simulink model "Copy_4_of_baseModel"  (R2019a)
settings: Solver=ode1  StartTime=0.0  StopTime=2.5  FixedStep=Ts_Power  RelTol=1e-3
PostLoadFcn:
  | %% Init for wind PnO models - global system parameters
  | OVERRIDE_SSN_MEMORY_LIMIT=1;
  | Ts=50e-6;
  | % Ts=50e-10;
  | Ts_Power=Ts;
  | Ts_Control=2*Ts;
  | freq = 50;
  | Fnom=freq;
  | Vac=400e3;
InitFcn:
  | %% Init for wind PnO models - global system parameters
  | OVERRIDE_SSN_MEMORY_LIMIT=1;
  | Ts=50e-6;
  | % Ts=50e-10;
  | Ts_Power=Ts;
  | Ts_Control=2*Ts;
  | freq = 50;
  | Fnom=freq;
  | Vac=225e3;
values from neighbouring files (symbols this model uses):
  ohl_posCap = (0.01e-006)*12    (= 1.2e-07)    [variable.m]
  ohl_posInd = (1.15e-3)/12    (= 9.58333333333e-05)    [variable.m]
  ohl_posR = 0.069/12    (= 0.00575)    [variable.m]
  ohl_zeroCap = (0.004e-006)*12    (= 4.8e-08)    [variable.m]
  ohl_zeroInd = (2.86e-3)/12    (= 0.000238333333333)    [variable.m]
  ohl_zeroR = 0.1725/12    (= 0.014375)    [variable.m]
  sub_posCap = sub_posCap*6    (= 9.6e-07)    [variable.m]
  sub_posInd = sub_posInd/6    (= 0.000233333333333)    [variable.m]
  sub_posR = sub_posR/6    (= 0.006)    [variable.m]
  sub_zeroCap = sub_zeroCap*6    (= 3.84e-07)    [variable.m]
  sub_zeroInd = sub_zeroInd/6    (= 0.000583333333333)    [variable.m]
  sub_zeroR = sub_zeroR/6    (= 0.015)    [variable.m]
  transfo_L1 = 0.05999374    [variable.m]
  transfo_L2 = 0.05999374    [variable.m]
  transfo_R1 = 0.000866667    [variable.m]
  transfo_R2 = 0.00086667    [variable.m]
undefined symbols (not defined in the file or in its folder): D1, D11, Delta, den, DiscIntNeverNeededParam, dx, find_system, gcbh, num, out_Buses, out_WindFarms, sps_rtmsupport
libraries: powerlib x172, simulink x80, powerlib_meascontrol x80, elements x52, eeSinusoidalMeasurement x44, simulink_extras x40, spsVIMeasurementModel x33, eePowerMeasurement x14
(part 10 of 22)

== system Copy_4_of_baseModel/SM_WT1/Differential Element 1/Main Protection (Current Differential)/Current Differential Protection for Phase C ==
  Ilocal : Inport
  Iremote : Inport  Port=2
  Icomp : Inport  Port=3
  " " : elements/   fo=Freq  window_size=40  harmonic=[1 2 3 4 5]
  " 1" : elements/   fo=Freq  window_size=40  harmonic=[1 2 3 4 5]
  Comparing Current at Master Station : Sum  Inputs=+-  SaturateOnIntegerOverflow=on  InputSameDT=on  OutDataTypeStr=Inherit: Same as first input
  Comparision Scheme : Subsystem
  DAB4 : Subsystem  mask(Data Adquisition Board){filter=off, approx=Bessel, order=2, numerator=[], denominator=[], freq=180, resdis=off, vertres=12, xmax=10, winsize=40, G=1.0, fs=Freq*40}
      mask prompts: filter "Disable Analog Filter"; approx "Filter approximation"; numerator "Free expression filter: numerator(descending order of s)"; denominator "Free expression filter: denominator:"; freq "Cut-off frequency"; resdis "Disable Vertical Resolution"; vertres "Vertical Resolution: No. of bits"; xmax "Vertical Resolution: signal range"; winsize "Window size"; G "Gain"; fs "Sampling frequency"
      mask help: Performs analog filtering, signal conditioning and sampling. A single signal is the input, a buffer with the signal samples is the output. The options include analog filter enable/disable switch, type, order and cut-off frequency of the analog filter, conditioning gain, sampling frequency, number of bits, the length of the buffer.
      mask init:
      | dab1
      mask TypeOptions approx: Bessel | Tschebyscheff | Butterworth | free expression
      mask TypeOptions order: 2 | 3 | 4
      mask TypeOptions vertres: 8 | 12 | 16
      mask Display: disp('DAB')
  DAB8 : Subsystem  mask(Data Adquisition Board){filter=off, approx=Bessel, order=2, numerator=[], denominator=[], freq=180, resdis=off, vertres=12, xmax=10, winsize=40, G=1.0, fs=Freq*40}
      mask prompts: filter "Disable Analog Filter"; approx "Filter approximation"; numerator "Free expression filter: numerator(descending order of s)"; denominator "Free expression filter: denominator:"; freq "Cut-off frequency"; resdis "Disable Vertical Resolution"; vertres "Vertical Resolution: No. of bits"; xmax "Vertical Resolution: signal range"; winsize "Window size"; G "Gain"; fs "Sampling frequency"
      mask help: Performs analog filtering, signal conditioning and sampling. A single signal is the input, a buffer with the signal samples is the output. The options include analog filter enable/disable switch, type, order and cut-off frequency of the analog filter, conditioning gain, sampling frequency, number of bits, the length of the buffer.
      mask init:
      | dab1
      mask TypeOptions approx: Bessel | Tschebyscheff | Butterworth | free expression
      mask TypeOptions order: 2 | 3 | 4
      mask TypeOptions vertres: 8 | 12 | 16
      mask Display: disp('DAB')
  Degrees to Radians : simulink_extras/Transformations/Degrees to Radians
  Degrees to Radians1 : simulink_extras/Transformations/Degrees to Radians
  Demux1 : Demux  Outputs=2
  Demux2 : Demux  Outputs=2
  Gain : Gain  SaturateOnIntegerOverflow=on  OutDataTypeStr=Inherit: Same as input  ParamDataTypeStr=Inherit: Same as input
  Gain1 : Gain  SaturateOnIntegerOverflow=on  OutDataTypeStr=Inherit: Same as input  ParamDataTypeStr=Inherit: Same as input
  Magnitude-Angle to Complex : MagnitudeAngleToComplex
  Magnitude-Angle to Complex1 : MagnitudeAngleToComplex
  Mux1 : Mux
  Mux2 : Mux
  Terminator1 : Terminator
  Terminator2 : Terminator
  Trip : Outport  InitialOutput=0  VectorParamsAs1DForOutWhenUnconnected=on
  wires:
  Gain1/1 -> Comparing Current at Master Station/2
  " 1"/2 -> Mux2/1
  " 1"/4 -> Mux2/3
  " 1"/3 -> Mux2/2
  Mux2/1 -> Terminator2/1
  Gain/1 -> DAB8/1(a)
  Iremote/1 -> Gain/1
  " 1"/1 -> Demux2/1
  DAB8/1(d) -> " 1"/1
  Magnitude-Angle to Complex1/1 -> Comparision Scheme/2(I_Master)
  Demux2/2 -> Degrees to Radians/1
  Degrees to Radians/1 -> Magnitude-Angle to Complex1/2
  Demux2/1 -> Magnitude-Angle to Complex1/1
  " "/5 -> Mux1/4
  " "/4 -> Mux1/3
  " "/3 -> Mux1/2
  " "/2 -> Mux1/1
  Mux1/1 -> Terminator1/1
  " "/1 -> Demux1/1
  Comparision Scheme/1(Pickup) -> Trip/1
  DAB4/1(d) -> " "/1
  Ilocal/1 -> DAB4/1(a)
  Magnitude-Angle to Complex/1 -> Comparing Current at Master Station/1
  Icomp/1 -> Gain1/1
  Demux1/2 -> Degrees to Radians1/1
  Degrees to Radians1/1 -> Magnitude-Angle to Complex/2
  Comparing Current at Master Station/1 -> Comparision Scheme/1(I_Slave)
  " 1"/5 -> Mux2/4
  Demux1/1 -> Magnitude-Angle to Complex/1

== system Copy_4_of_baseModel/SM_WT1/Differential Element 2/Main Protection (Current Differential)/Charging Current Compensation phase A ==
  VA : Inport
  VB : Inport  Port=2
  VC : Inport  Port=3
  " 5" : elements/   fo=Freq  window_size=40  harmonic=[1 2 3 4 5]
  " 6" : elements/   fo=Freq  window_size=40  harmonic=[1 2 3 4 5]
  " 7" : elements/   fo=Freq  window_size=40  harmonic=[1 2 3 4 5]
  *2 : Gain  Gain=2  SaturateOnIntegerOverflow=on  OutDataTypeStr=Inherit: Same as input  ParamDataTypeStr=Inherit: Same as input
  Compensating Current : Sum  SaturateOnIntegerOverflow=on  InputSameDT=on  OutDataTypeStr=Inherit: Same as first input
  Cpg : Gain  Gain=Cpg  SaturateOnIntegerOverflow=on  OutDataTypeStr=Inherit: Same as input  ParamDataTypeStr=Inherit: Same as input
  Cpp : Gain  Gain=Cpp  SaturateOnIntegerOverflow=on  OutDataTypeStr=Inherit: Same as input  ParamDataTypeStr=Inherit: Same as input
  DAB5 : Subsystem  mask(Data Adquisition Board){filter=off, approx=Bessel, order=2, numerator=[], denominator=[], freq=180, resdis=off, vertres=12, xmax=10, winsize=40, G=1.0, fs=Freq*40}
      mask prompts: filter "Disable Analog Filter"; approx "Filter approximation"; numerator "Free expression filter: numerator(descending order of s)"; denominator "Free expression filter: denominator:"; freq "Cut-off frequency"; resdis "Disable Vertical Resolution"; vertres "Vertical Resolution: No. of bits"; xmax "Vertical Resolution: signal range"; winsize "Window size"; G "Gain"; fs "Sampling frequency"
      mask help: Performs analog filtering, signal conditioning and sampling. A single signal is the input, a buffer with the signal samples is the output. The options include analog filter enable/disable switch, type, order and cut-off frequency of the analog filter, conditioning gain, sampling frequency, number of bits, the length of the buffer.
      mask init:
      | dab1
      mask TypeOptions approx: Bessel | Tschebyscheff | Butterworth | free expression
      mask TypeOptions order: 2 | 3 | 4
      mask TypeOptions vertres: 8 | 12 | 16
      mask Display: disp('DAB')
  DAB6 : Subsystem  mask(Data Adquisition Board){filter=off, approx=Bessel, order=2, numerator=[], denominator=[], freq=180, resdis=off, vertres=12, xmax=10, winsize=40, G=1.0, fs=Freq*40}
      mask prompts: filter "Disable Analog Filter"; approx "Filter approximation"; numerator "Free expression filter: numerator(descending order of s)"; denominator "Free expression filter: denominator:"; freq "Cut-off frequency"; resdis "Disable Vertical Resolution"; vertres "Vertical Resolution: No. of bits"; xmax "Vertical Resolution: signal range"; winsize "Window size"; G "Gain"; fs "Sampling frequency"
      mask help: Performs analog filtering, signal conditioning and sampling. A single signal is the input, a buffer with the signal samples is the output. The options include analog filter enable/disable switch, type, order and cut-off frequency of the analog filter, conditioning gain, sampling frequency, number of bits, the length of the buffer.
      mask init:
      | dab1
      mask TypeOptions approx: Bessel | Tschebyscheff | Butterworth | free expression
      mask TypeOptions order: 2 | 3 | 4
      mask TypeOptions vertres: 8 | 12 | 16
      mask Display: disp('DAB')
  DAB7 : Subsystem  mask(Data Adquisition Board){filter=off, approx=Bessel, order=2, numerator=[], denominator=[], freq=180, resdis=off, vertres=12, xmax=10, winsize=40, G=1.0, fs=Freq*40}
      mask prompts: filter "Disable Analog Filter"; approx "Filter approximation"; numerator "Free expression filter: numerator(descending order of s)"; denominator "Free expression filter: denominator:"; freq "Cut-off frequency"; resdis "Disable Vertical Resolution"; vertres "Vertical Resolution: No. of bits"; xmax "Vertical Resolution: signal range"; winsize "Window size"; G "Gain"; fs "Sampling frequency"
      mask help: Performs analog filtering, signal conditioning and sampling. A single signal is the input, a buffer with the signal samples is the output. The options include analog filter enable/disable switch, type, order and cut-off frequency of the analog filter, conditioning gain, sampling frequency, number of bits, the length of the buffer.
      mask init:
      | dab1
      mask TypeOptions approx: Bessel | Tschebyscheff | Butterworth | free expression
      mask TypeOptions order: 2 | 3 | 4
      mask TypeOptions vertres: 8 | 12 | 16
      mask Display: disp('DAB')
  Degrees to Radians1 : simulink_extras/Transformations/Degrees to Radians
  Degrees to Radians2 : simulink_extras/Transformations/Degrees to Radians
  Degrees to Radians3 : simulink_extras/Transformations/Degrees to Radians
  Demux : Demux  Outputs=2
  Demux1 : Demux  Outputs=2
  Demux2 : Demux  Outputs=2
  Derivative : Derivative
  Derivative1 : Derivative
  Derivative2 : Derivative
  Magnitude-Angle to Complex : MagnitudeAngleToComplex
  Magnitude-Angle to Complex1 : MagnitudeAngleToComplex
  Magnitude-Angle to Complex2 : MagnitudeAngleToComplex
  Mux : Mux  Inputs=12
  Terminator : Terminator
  sum : Sum  Inputs=+--  SaturateOnIntegerOverflow=on  InputSameDT=on  OutDataTypeStr=Inherit: Same as first input
  Icomp : Outport  VectorParamsAs1DForOutWhenUnconnected=on
  wires:
  " 5"/1 -> Demux2/1
  Demux1/2 -> Degrees to Radians2/1
  Demux1/1 -> Magnitude-Angle to Complex1/1
  " 7"/1 -> Demux/1
  Derivative1/1 -> DAB6/1(a)
  DAB6/1(d) -> " 6"/1
  " 6"/1 -> Demux1/1
  VB/1 -> Derivative1/1
  Mux/1 -> Terminator/1
  " 5"/5 -> Mux/4
  Derivative/1 -> DAB5/1(a)
  DAB5/1(d) -> " 5"/1
  Cpg/1 -> Compensating Current/1
  VA/1 -> Derivative/1
  " 5"/2 -> Mux/1
  " 5"/3 -> Mux/2
  " 5"/4 -> Mux/3
  sum/1 -> Cpp/1
  Compensating Current/1 -> Icomp/1
  *2/1 -> sum/1
  Cpp/1 -> Compensating Current/2
  Derivative2/1 -> DAB7/1(a)
  DAB7/1(d) -> " 7"/1
  VC/1 -> Derivative2/1
  " 7"/2 -> Mux/9
  " 7"/3 -> Mux/10
  " 7"/4 -> Mux/11
  " 7"/5 -> Mux/12
  " 6"/2 -> Mux/5
  " 6"/3 -> Mux/6
  " 6"/4 -> Mux/7
  " 6"/5 -> Mux/8
  Demux2/1 -> Magnitude-Angle to Complex/1
  Magnitude-Angle to Complex/1 -> *2/1, Cpg/1
  Magnitude-Angle to Complex1/1 -> sum/2
  Demux/1 -> Magnitude-Angle to Complex2/1
  Magnitude-Angle to Complex2/1 -> sum/3
  Demux/2 -> Degrees to Radians1/1
  Degrees to Radians1/1 -> Magnitude-Angle to Complex2/2
  Degrees to Radians2/1 -> Magnitude-Angle to Complex1/2
  Demux2/2 -> Degrees to Radians3/1
  Degrees to Radians3/1 -> Magnitude-Angle to Complex/2

== system Copy_4_of_baseModel/SM_WT1/Differential Element 2/Main Protection (Current Differential)/Charging Current Compensation phase B ==
  VA : Inport
  VB : Inport  Port=2
  VC : Inport  Port=3
  " 5" : elements/   fo=Freq  window_size=40  harmonic=[1 2 3 4 5]
  " 6" : elements/   fo=Freq  window_size=40  harmonic=[1 2 3 4 5]
  " 7" : elements/   fo=Freq  window_size=40  harmonic=[1 2 3 4 5]
  *2 : Gain  Gain=2  SaturateOnIntegerOverflow=on  OutDataTypeStr=Inherit: Same as input  ParamDataTypeStr=Inherit: Same as input
  Compensating Current : Sum  SaturateOnIntegerOverflow=on  InputSameDT=on  OutDataTypeStr=Inherit: Same as first input
  Cpg : Gain  Gain=Cpg  SaturateOnIntegerOverflow=on  OutDataTypeStr=Inherit: Same as input  ParamDataTypeStr=Inherit: Same as input
  Cpp : Gain  Gain=Cpp  SaturateOnIntegerOverflow=on  OutDataTypeStr=Inherit: Same as input  ParamDataTypeStr=Inherit: Same as input
  DAB5 : Subsystem  mask(Data Adquisition Board){filter=off, approx=Bessel, order=2, numerator=[], denominator=[], freq=180, resdis=off, vertres=12, xmax=10, winsize=40, G=1.0, fs=Freq*40}
      mask prompts: filter "Disable Analog Filter"; approx "Filter approximation"; numerator "Free expression filter: numerator(descending order of s)"; denominator "Free expression filter: denominator:"; freq "Cut-off frequency"; resdis "Disable Vertical Resolution"; vertres "Vertical Resolution: No. of bits"; xmax "Vertical Resolution: signal range"; winsize "Window size"; G "Gain"; fs "Sampling frequency"
      mask help: Performs analog filtering, signal conditioning and sampling. A single signal is the input, a buffer with the signal samples is the output. The options include analog filter enable/disable switch, type, order and cut-off frequency of the analog filter, conditioning gain, sampling frequency, number of bits, the length of the buffer.
      mask init:
      | dab1
      mask TypeOptions approx: Bessel | Tschebyscheff | Butterworth | free expression
      mask TypeOptions order: 2 | 3 | 4
      mask TypeOptions vertres: 8 | 12 | 16
      mask Display: disp('DAB')
  DAB6 : Subsystem  mask(Data Adquisition Board){filter=off, approx=Bessel, order=2, numerator=[], denominator=[], freq=180, resdis=off, vertres=12, xmax=10, winsize=40, G=1.0, fs=Freq*40}
      mask prompts: filter "Disable Analog Filter"; approx "Filter approximation"; numerator "Free expression filter: numerator(descending order of s)"; denominator "Free expression filter: denominator:"; freq "Cut-off frequency"; resdis "Disable Vertical Resolution"; vertres "Vertical Resolution: No. of bits"; xmax "Vertical Resolution: signal range"; winsize "Window size"; G "Gain"; fs "Sampling frequency"
      mask help: Performs analog filtering, signal conditioning and sampling. A single signal is the input, a buffer with the signal samples is the output. The options include analog filter enable/disable switch, type, order and cut-off frequency of the analog filter, conditioning gain, sampling frequency, number of bits, the length of the buffer.
      mask init:
      | dab1
      mask TypeOptions approx: Bessel | Tschebyscheff | Butterworth | free expression
      mask TypeOptions order: 2 | 3 | 4
      mask TypeOptions vertres: 8 | 12 | 16
      mask Display: disp('DAB')
  DAB7 : Subsystem  mask(Data Adquisition Board){filter=off, approx=Bessel, order=2, numerator=[], denominator=[], freq=180, resdis=off, vertres=12, xmax=10, winsize=40, G=1.0, fs=Freq*40}
      mask prompts: filter "Disable Analog Filter"; approx "Filter approximation"; numerator "Free expression filter: numerator(descending order of s)"; denominator "Free expression filter: denominator:"; freq "Cut-off frequency"; resdis "Disable Vertical Resolution"; vertres "Vertical Resolution: No. of bits"; xmax "Vertical Resolution: signal range"; winsize "Window size"; G "Gain"; fs "Sampling frequency"
      mask help: Performs analog filtering, signal conditioning and sampling. A single signal is the input, a buffer with the signal samples is the output. The options include analog filter enable/disable switch, type, order and cut-off frequency of the analog filter, conditioning gain, sampling frequency, number of bits, the length of the buffer.
      mask init:
      | dab1
      mask TypeOptions approx: Bessel | Tschebyscheff | Butterworth | free expression
      mask TypeOptions order: 2 | 3 | 4
      mask TypeOptions vertres: 8 | 12 | 16
      mask Display: disp('DAB')
  Degrees to Radians1 : simulink_extras/Transformations/Degrees to Radians
  Degrees to Radians2 : simulink_extras/Transformations/Degrees to Radians
  Degrees to Radians3 : simulink_extras/Transformations/Degrees to Radians
  Demux : Demux  Outputs=2
  Demux1 : Demux  Outputs=2
  Demux2 : Demux  Outputs=2
  Derivative : Derivative
  Derivative1 : Derivative
  Derivative2 : Derivative
  Magnitude-Angle to Complex : MagnitudeAngleToComplex
  Magnitude-Angle to Complex1 : MagnitudeAngleToComplex
  Magnitude-Angle to Complex2 : MagnitudeAngleToComplex
  Mux : Mux  Inputs=12
  Terminator : Terminator
  sum : Sum  Inputs=+--  SaturateOnIntegerOverflow=on  InputSameDT=on  OutDataTypeStr=Inherit: Same as first input
  Icomp : Outport  VectorParamsAs1DForOutWhenUnconnected=on
  wires:
  VA/1 -> Derivative1/1
  VB/1 -> Derivative/1
  " 5"/1 -> Demux2/1
  Demux1/2 -> Degrees to Radians2/1
  Demux1/1 -> Magnitude-Angle to Complex1/1
  " 7"/1 -> Demux/1
  Derivative1/1 -> DAB6/1(a)
  DAB6/1(d) -> " 6"/1
  " 6"/1 -> Demux1/1
  Mux/1 -> Terminator/1
  " 5"/5 -> Mux/4
  Derivative/1 -> DAB5/1(a)
  DAB5/1(d) -> " 5"/1
  Cpg/1 -> Compensating Current/1
  " 5"/2 -> Mux/1
  " 5"/3 -> Mux/2
  " 5"/4 -> Mux/3
  sum/1 -> Cpp/1
  Compensating Current/1 -> Icomp/1
  *2/1 -> sum/1
  Cpp/1 -> Compensating Current/2
  Derivative2/1 -> DAB7/1(a)
  DAB7/1(d) -> " 7"/1
  VC/1 -> Derivative2/1
  " 7"/2 -> Mux/9
  " 7"/3 -> Mux/10
  " 7"/4 -> Mux/11
  " 7"/5 -> Mux/12
  " 6"/2 -> Mux/5
  " 6"/3 -> Mux/6
  " 6"/4 -> Mux/7
  " 6"/5 -> Mux/8
  Demux2/1 -> Magnitude-Angle to Complex/1
  Magnitude-Angle to Complex/1 -> *2/1, Cpg/1
  Magnitude-Angle to Complex1/1 -> sum/2
  Demux/1 -> Magnitude-Angle to Complex2/1
  Magnitude-Angle to Complex2/1 -> sum/3
  Demux/2 -> Degrees to Radians1/1
  Degrees to Radians1/1 -> Magnitude-Angle to Complex2/2
  Degrees to Radians2/1 -> Magnitude-Angle to Complex1/2
  Demux2/2 -> Degrees to Radians3/1
  Degrees to Radians3/1 -> Magnitude-Angle to Complex/2

== system Copy_4_of_baseModel/SM_WT1/Differential Element 2/Main Protection (Current Differential)/Charging Current Compensation phase C ==
  VA : Inport
  VB : Inport  Port=2
  VC : Inport  Port=3
  " 5" : elements/   fo=Freq  window_size=40  harmonic=[1 2 3 4 5]
  " 6" : elements/   fo=Freq  window_size=40  harmonic=[1 2 3 4 5]
  " 7" : elements/   fo=Freq  window_size=40  harmonic=[1 2 3 4 5]
  *2 : Gain  Gain=2  SaturateOnIntegerOverflow=on  OutDataTypeStr=Inherit: Same as input  ParamDataTypeStr=Inherit: Same as input
  Compensating Current : Sum  SaturateOnIntegerOverflow=on  InputSameDT=on  OutDataTypeStr=Inherit: Same as first input
  Cpg : Gain  Gain=Cpg  SaturateOnIntegerOverflow=on  OutDataTypeStr=Inherit: Same as input  ParamDataTypeStr=Inherit: Same as input
  Cpp : Gain  Gain=Cpp  SaturateOnIntegerOverflow=on  OutDataTypeStr=Inherit: Same as input  ParamDataTypeStr=Inherit: Same as input
  DAB5 : Subsystem  mask(Data Adquisition Board){filter=off, approx=Bessel, order=2, numerator=[], denominator=[], freq=180, resdis=off, vertres=12, xmax=10, winsize=40, G=1.0, fs=Freq*40}
      mask prompts: filter "Disable Analog Filter"; approx "Filter approximation"; numerator "Free expression filter: numerator(descending order of s)"; denominator "Free expression filter: denominator:"; freq "Cut-off frequency"; resdis "Disable Vertical Resolution"; vertres "Vertical Resolution: No. of bits"; xmax "Vertical Resolution: signal range"; winsize "Window size"; G "Gain"; fs "Sampling frequency"
      mask help: Performs analog filtering, signal conditioning and sampling. A single signal is the input, a buffer with the signal samples is the output. The options include analog filter enable/disable switch, type, order and cut-off frequency of the analog filter, conditioning gain, sampling frequency, number of bits, the length of the buffer.
      mask init:
      | dab1
      mask TypeOptions approx: Bessel | Tschebyscheff | Butterworth | free expression
      mask TypeOptions order: 2 | 3 | 4
      mask TypeOptions vertres: 8 | 12 | 16
      mask Display: disp('DAB')
  DAB6 : Subsystem  mask(Data Adquisition Board){filter=off, approx=Bessel, order=2, numerator=[], denominator=[], freq=180, resdis=off, vertres=12, xmax=10, winsize=40, G=1.0, fs=Freq*40}
      mask prompts: filter "Disable Analog Filter"; approx "Filter approximation"; numerator "Free expression filter: numerator(descending order of s)"; denominator "Free expression filter: denominator:"; freq "Cut-off frequency"; resdis "Disable Vertical Resolution"; vertres "Vertical Resolution: No. of bits"; xmax "Vertical Resolution: signal range"; winsize "Window size"; G "Gain"; fs "Sampling frequency"
      mask help: Performs analog filtering, signal conditioning and sampling. A single signal is the input, a buffer with the signal samples is the output. The options include analog filter enable/disable switch, type, order and cut-off frequency of the analog filter, conditioning gain, sampling frequency, number of bits, the length of the buffer.
      mask init:
      | dab1
      mask TypeOptions approx: Bessel | Tschebyscheff | Butterworth | free expression
      mask TypeOptions order: 2 | 3 | 4
      mask TypeOptions vertres: 8 | 12 | 16
      mask Display: disp('DAB')
  DAB7 : Subsystem  mask(Data Adquisition Board){filter=off, approx=Bessel, order=2, numerator=[], denominator=[], freq=180, resdis=off, vertres=12, xmax=10, winsize=40, G=1.0, fs=Freq*40}
      mask prompts: filter "Disable Analog Filter"; approx "Filter approximation"; numerator "Free expression filter: numerator(descending order of s)"; denominator "Free expression filter: denominator:"; freq "Cut-off frequency"; resdis "Disable Vertical Resolution"; vertres "Vertical Resolution: No. of bits"; xmax "Vertical Resolution: signal range"; winsize "Window size"; G "Gain"; fs "Sampling frequency"
      mask help: Performs analog filtering, signal conditioning and sampling. A single signal is the input, a buffer with the signal samples is the output. The options include analog filter enable/disable switch, type, order and cut-off frequency of the analog filter, conditioning gain, sampling frequency, number of bits, the length of the buffer.
      mask init:
      | dab1
      mask TypeOptions approx: Bessel | Tschebyscheff | Butterworth | free expression
      mask TypeOptions order: 2 | 3 | 4
      mask TypeOptions vertres: 8 | 12 | 16
      mask Display: disp('DAB')
  Degrees to Radians1 : simulink_extras/Transformations/Degrees to Radians
  Degrees to Radians2 : simulink_extras/Transformations/Degrees to Radians
  Degrees to Radians3 : simulink_extras/Transformations/Degrees to Radians
  Demux : Demux  Outputs=2
  Demux1 : Demux  Outputs=2
  Demux2 : Demux  Outputs=2
  Derivative : Derivative
  Derivative1 : Derivative
  Derivative2 : Derivative
  Magnitude-Angle to Complex : MagnitudeAngleToComplex
  Magnitude-Angle to Complex1 : MagnitudeAngleToComplex
  Magnitude-Angle to Complex2 : MagnitudeAngleToComplex
  Mux : Mux  Inputs=12
  Terminator : Terminator
  sum : Sum  Inputs=+--  SaturateOnIntegerOverflow=on  InputSameDT=on  OutDataTypeStr=Inherit: Same as first input
  Icomp : Outport  VectorParamsAs1DForOutWhenUnconnected=on
  wires:
  VA/1 -> Derivative2/1
  VC/1 -> Derivative/1
  " 5"/1 -> Demux2/1
  Demux1/2 -> Degrees to Radians2/1
  Demux1/1 -> Magnitude-Angle to Complex1/1
  " 7"/1 -> Demux/1
  Derivative1/1 -> DAB6/1(a)
  DAB6/1(d) -> " 6"/1
  " 6"/1 -> Demux1/1
  VB/1 -> Derivative1/1
  Mux/1 -> Terminator/1
  " 5"/5 -> Mux/4
  Derivative/1 -> DAB5/1(a)
  DAB5/1(d) -> " 5"/1
  Cpg/1 -> Compensating Current/1
  " 5"/2 -> Mux/1
  " 5"/3 -> Mux/2
  " 5"/4 -> Mux/3
  sum/1 -> Cpp/1
  Compensating Current/1 -> Icomp/1
  *2/1 -> sum/1
  Cpp/1 -> Compensating Current/2
  Derivative2/1 -> DAB7/1(a)
  DAB7/1(d) -> " 7"/1
  " 7"/2 -> Mux/9
  " 7"/3 -> Mux/10
  " 7"/4 -> Mux/11
  " 7"/5 -> Mux/12
  " 6"/2 -> Mux/5
  " 6"/3 -> Mux/6
  " 6"/4 -> Mux/7
  " 6"/5 -> Mux/8
  Demux2/1 -> Magnitude-Angle to Complex/1
  Magnitude-Angle to Complex/1 -> *2/1, Cpg/1
  Magnitude-Angle to Complex1/1 -> sum/2
  Demux/1 -> Magnitude-Angle to Complex2/1
  Magnitude-Angle to Complex2/1 -> sum/3
  Demux/2 -> Degrees to Radians1/1
  Degrees to Radians1/1 -> Magnitude-Angle to Complex2/2
  Degrees to Radians2/1 -> Magnitude-Angle to Complex1/2
  Demux2/2 -> Degrees to Radians3/1
  Degrees to Radians3/1 -> Magnitude-Angle to Complex/2

== system Copy_4_of_baseModel/SM_WT1/Differential Element 2/Main Protection (Current Differential)/Current Differential Protection for Phase A ==
  Ilocal : Inport
  Iremote : Inport  Port=2
  Icomp : Inport  Port=3
  " " : elements/   fo=Freq  window_size=40  harmonic=[1 2 3 4 5]
  " 1" : elements/   fo=Freq  window_size=40  harmonic=[1 2 3 4 5]
  Comparing Current at Master Station : Sum  Inputs=+-  SaturateOnIntegerOverflow=on  InputSameDT=on  OutDataTypeStr=Inherit: Same as first input
  Comparision Scheme : Subsystem
  DAB4 : Subsystem  mask(Data Adquisition Board){filter=off, approx=Bessel, order=2, numerator=[], denominator=[], freq=180, resdis=off, vertres=12, xmax=10, winsize=40, G=1.0, fs=Freq*40}
      mask prompts: filter "Disable Analog Filter"; approx "Filter approximation"; numerator "Free expression filter: numerator(descending order of s)"; denominator "Free expression filter: denominator:"; freq "Cut-off frequency"; resdis "Disable Vertical Resolution"; vertres "Vertical Resolution: No. of bits"; xmax "Vertical Resolution: signal range"; winsize "Window size"; G "Gain"; fs "Sampling frequency"
      mask help: Performs analog filtering, signal conditioning and sampling. A single signal is the input, a buffer with the signal samples is the output. The options include analog filter enable/disable switch, type, order and cut-off frequency of the analog filter, conditioning gain, sampling frequency, number of bits, the length of the buffer.
      mask init:
      | dab1
      mask TypeOptions approx: Bessel | Tschebyscheff | Butterworth | free expression
      mask TypeOptions order: 2 | 3 | 4
      mask TypeOptions vertres: 8 | 12 | 16
      mask Display: disp('DAB')
  DAB8 : Subsystem  mask(Data Adquisition Board){filter=off, approx=Bessel, order=2, numerator=[], denominator=[], freq=180, resdis=off, vertres=12, xmax=10, winsize=40, G=1.0, fs=Freq*40}
      mask prompts: filter "Disable Analog Filter"; approx "Filter approximation"; numerator "Free expression filter: numerator(descending order of s)"; denominator "Free expression filter: denominator:"; freq "Cut-off frequency"; resdis "Disable Vertical Resolution"; vertres "Vertical Resolution: No. of bits"; xmax "Vertical Resolution: signal range"; winsize "Window size"; G "Gain"; fs "Sampling frequency"
      mask help: Performs analog filtering, signal conditioning and sampling. A single signal is the input, a buffer with the signal samples is the output. The options include analog filter enable/disable switch, type, order and cut-off frequency of the analog filter, conditioning gain, sampling frequency, number of bits, the length of the buffer.
      mask init:
      | dab1
      mask TypeOptions approx: Bessel | Tschebyscheff | Butterworth | free expression
      mask TypeOptions order: 2 | 3 | 4
      mask TypeOptions vertres: 8 | 12 | 16
      mask Display: disp('DAB')
  Degrees to Radians : simulink_extras/Transformations/Degrees to Radians
  Degrees to Radians1 : simulink_extras/Transformations/Degrees to Radians
  Demux1 : Demux  Outputs=2
  Demux2 : Demux  Outputs=2
  Gain : Gain  SaturateOnIntegerOverflow=on  OutDataTypeStr=Inherit: Same as input  ParamDataTypeStr=Inherit: Same as input
  Gain1 : Gain  SaturateOnIntegerOverflow=on  OutDataTypeStr=Inherit: Same as input  ParamDataTypeStr=Inherit: Same as input
  Magnitude-Angle to Complex : MagnitudeAngleToComplex
  Magnitude-Angle to Complex1 : MagnitudeAngleToComplex
  Mux1 : Mux
  Mux2 : Mux
  Terminator1 : Terminator
  Terminator2 : Terminator
  Trip : Outport  InitialOutput=0  VectorParamsAs1DForOutWhenUnconnected=on
  wires:
  Gain1/1 -> Comparing Current at Master Station/2
  " 1"/2 -> Mux2/1
  " 1"/4 -> Mux2/3
  " 1"/3 -> Mux2/2
  Mux2/1 -> Terminator2/1
  Gain/1 -> DAB8/1(a)
  Iremote/1 -> Gain/1
  " 1"/1 -> Demux2/1
  DAB8/1(d) -> " 1"/1
  Magnitude-Angle to Complex1/1 -> Comparision Scheme/2(I_Master)
  Demux2/2 -> Degrees to Radians/1
  Degrees to Radians/1 -> Magnitude-Angle to Complex1/2
  Demux2/1 -> Magnitude-Angle to Complex1/1
  " "/5 -> Mux1/4
  " "/4 -> Mux1/3
  " "/3 -> Mux1/2
  " "/2 -> Mux1/1
  Mux1/1 -> Terminator1/1
  " "/1 -> Demux1/1
  Comparision Scheme/1(Pickup) -> Trip/1
  DAB4/1(d) -> " "/1
  Ilocal/1 -> DAB4/1(a)
  Magnitude-Angle to Complex/1 -> Comparing Current at Master Station/1
  Icomp/1 -> Gain1/1
  Demux1/2 -> Degrees to Radians1/1
  Degrees to Radians1/1 -> Magnitude-Angle to Complex/2
  Comparing Current at Master Station/1 -> Comparision Scheme/1(I_Slave)
  " 1"/5 -> Mux2/4
  Demux1/1 -> Magnitude-Angle to Complex/1

== system Copy_4_of_baseModel/SM_WT1/Differential Element 2/Main Protection (Current Differential)/Current Differential Protection for Phase B ==
  Ilocal : Inport
  Iremote : Inport  Port=2
  Icomp : Inport  Port=3
  " " : elements/   fo=Freq  window_size=40  harmonic=[1 2 3 4 5]
  " 1" : elements/   fo=Freq  window_size=40  harmonic=[1 2 3 4 5]
  Comparing Current at Master Station : Sum  Inputs=+-  SaturateOnIntegerOverflow=on  InputSameDT=on  OutDataTypeStr=Inherit: Same as first input
  Comparision Scheme : Subsystem
  DAB4 : Subsystem  mask(Data Adquisition Board){filter=off, approx=Bessel, order=2, numerator=[], denominator=[], freq=180, resdis=off, vertres=12, xmax=10, winsize=40, G=1.0, fs=Freq*40}
      mask prompts: filter "Disable Analog Filter"; approx "Filter approximation"; numerator "Free expression filter: numerator(descending order of s)"; denominator "Free expression filter: denominator:"; freq "Cut-off frequency"; resdis "Disable Vertical Resolution"; vertres "Vertical Resolution: No. of bits"; xmax "Vertical Resolution: signal range"; winsize "Window size"; G "Gain"; fs "Sampling frequency"
      mask help: Performs analog filtering, signal conditioning and sampling. A single signal is the input, a buffer with the signal samples is the output. The options include analog filter enable/disable switch, type, order and cut-off frequency of the analog filter, conditioning gain, sampling frequency, number of bits, the length of the buffer.
      mask init:
      | dab1
      mask TypeOptions approx: Bessel | Tschebyscheff | Butterworth | free expression
      mask TypeOptions order: 2 | 3 | 4
      mask TypeOptions vertres: 8 | 12 | 16
      mask Display: disp('DAB')
  DAB8 : Subsystem  mask(Data Adquisition Board){filter=off, approx=Bessel, order=2, numerator=[], denominator=[], freq=180, resdis=off, vertres=12, xmax=10, winsize=40, G=1.0, fs=Freq*40}
      mask prompts: filter "Disable Analog Filter"; approx "Filter approximation"; numerator "Free expression filter: numerator(descending order of s)"; denominator "Free expression filter: denominator:"; freq "Cut-off frequency"; resdis "Disable Vertical Resolution"; vertres "Vertical Resolution: No. of bits"; xmax "Vertical Resolution: signal range"; winsize "Window size"; G "Gain"; fs "Sampling frequency"
      mask help: Performs analog filtering, signal conditioning and sampling. A single signal is the input, a buffer with the signal samples is the output. The options include analog filter enable/disable switch, type, order and cut-off frequency of the analog filter, conditioning gain, sampling frequency, number of bits, the length of the buffer.
      mask init:
      | dab1
      mask TypeOptions approx: Bessel | Tschebyscheff | Butterworth | free expression
      mask TypeOptions order: 2 | 3 | 4
      mask TypeOptions vertres: 8 | 12 | 16
      mask Display: disp('DAB')
  Degrees to Radians : simulink_extras/Transformations/Degrees to Radians
  Degrees to Radians1 : simulink_extras/Transformations/Degrees to Radians
  Demux1 : Demux  Outputs=2
  Demux2 : Demux  Outputs=2
  Gain : Gain  SaturateOnIntegerOverflow=on  OutDataTypeStr=Inherit: Same as input  ParamDataTypeStr=Inherit: Same as input
  Gain1 : Gain  SaturateOnIntegerOverflow=on  OutDataTypeStr=Inherit: Same as input  ParamDataTypeStr=Inherit: Same as input
  Magnitude-Angle to Complex : MagnitudeAngleToComplex
  Magnitude-Angle to Complex1 : MagnitudeAngleToComplex
  Mux1 : Mux
  Mux2 : Mux
  Terminator1 : Terminator
  Terminator2 : Terminator
  Trip : Outport  InitialOutput=0  VectorParamsAs1DForOutWhenUnconnected=on
  wires:
  Gain1/1 -> Comparing Current at Master Station/2
  Demux1/1 -> Magnitude-Angle to Complex/1
  " 1"/5 -> Mux2/4
  Comparing Current at Master Station/1 -> Comparision Scheme/1(I_Slave)
  Degrees to Radians1/1 -> Magnitude-Angle to Complex/2
  Demux1/2 -> Degrees to Radians1/1
  Icomp/1 -> Gain1/1
  Magnitude-Angle to Complex/1 -> Comparing Current at Master Station/1
  Ilocal/1 -> DAB4/1(a)
  DAB4/1(d) -> " "/1
  Comparision Scheme/1(Pickup) -> Trip/1
  " "/1 -> Demux1/1
  Mux1/1 -> Terminator1/1
  " "/2 -> Mux1/1
  " "/3 -> Mux1/2
  " "/4 -> Mux1/3
  " "/5 -> Mux1/4
  Demux2/1 -> Magnitude-Angle to Complex1/1
  Degrees to Radians/1 -> Magnitude-Angle to Complex1/2
  Demux2/2 -> Degrees to Radians/1
  Magnitude-Angle to Complex1/1 -> Comparision Scheme/2(I_Master)
  DAB8/1(d) -> " 1"/1
  " 1"/1 -> Demux2/1
  Iremote/1 -> Gain/1
  Gain/1 -> DAB8/1(a)
  Mux2/1 -> Terminator2/1
  " 1"/3 -> Mux2/2
  " 1"/4 -> Mux2/3
  " 1"/2 -> Mux2/1

== system Copy_4_of_baseModel/SM_WT1/Differential Element 2/Main Protection (Current Differential)/Current Differential Protection for Phase C ==
  Ilocal : Inport
  Iremote : Inport  Port=2
  Icomp : Inport  Port=3
  " " : elements/   fo=Freq  window_size=40  harmonic=[1 2 3 4 5]
  " 1" : elements/   fo=Freq  window_size=40  harmonic=[1 2 3 4 5]
  Comparing Current at Master Station : Sum  Inputs=+-  SaturateOnIntegerOverflow=on  InputSameDT=on  OutDataTypeStr=Inherit: Same as first input
  Comparision Scheme : Subsystem
  DAB4 : Subsystem  mask(Data Adquisition Board){filter=off, approx=Bessel, order=2, numerator=[], denominator=[], freq=180, resdis=off, vertres=12, xmax=10, winsize=40, G=1.0, fs=Freq*40}
      mask prompts: filter "Disable Analog Filter"; approx "Filter approximation"; numerator "Free expression filter: numerator(descending order of s)"; denominator "Free expression filter: denominator:"; freq "Cut-off frequency"; resdis "Disable Vertical Resolution"; vertres "Vertical Resolution: No. of bits"; xmax "Vertical Resolution: signal range"; winsize "Window size"; G "Gain"; fs "Sampling frequency"
      mask help: Performs analog filtering, signal conditioning and sampling. A single signal is the input, a buffer with the signal samples is the output. The options include analog filter enable/disable switch, type, order and cut-off frequency of the analog filter, conditioning gain, sampling frequency, number of bits, the length of the buffer.
      mask init:
      | dab1
      mask TypeOptions approx: Bessel | Tschebyscheff | Butterworth | free expression
      mask TypeOptions order: 2 | 3 | 4
      mask TypeOptions vertres: 8 | 12 | 16
      mask Display: disp('DAB')
  DAB8 : Subsystem  mask(Data Adquisition Board){filter=off, approx=Bessel, order=2, numerator=[], denominator=[], freq=180, resdis=off, vertres=12, xmax=10, winsize=40, G=1.0, fs=Freq*40}
      mask prompts: filter "Disable Analog Filter"; approx "Filter approximation"; numerator "Free expression filter: numerator(descending order of s)"; denominator "Free expression filter: denominator:"; freq "Cut-off frequency"; resdis "Disable Vertical Resolution"; vertres "Vertical Resolution: No. of bits"; xmax "Vertical Resolution: signal range"; winsize "Window size"; G "Gain"; fs "Sampling frequency"
      mask help: Performs analog filtering, signal conditioning and sampling. A single signal is the input, a buffer with the signal samples is the output. The options include analog filter enable/disable switch, type, order and cut-off frequency of the analog filter, conditioning gain, sampling frequency, number of bits, the length of the buffer.
      mask init:
      | dab1
      mask TypeOptions approx: Bessel | Tschebyscheff | Butterworth | free expression
      mask TypeOptions order: 2 | 3 | 4
      mask TypeOptions vertres: 8 | 12 | 16
      mask Display: disp('DAB')
  Degrees to Radians : simulink_extras/Transformations/Degrees to Radians
  Degrees to Radians1 : simulink_extras/Transformations/Degrees to Radians
  Demux1 : Demux  Outputs=2
  Demux2 : Demux  Outputs=2
  Gain : Gain  SaturateOnIntegerOverflow=on  OutDataTypeStr=Inherit: Same as input  ParamDataTypeStr=Inherit: Same as input
  Gain1 : Gain  SaturateOnIntegerOverflow=on  OutDataTypeStr=Inherit: Same as input  ParamDataTypeStr=Inherit: Same as input
  Magnitude-Angle to Complex : MagnitudeAngleToComplex
  Magnitude-Angle to Complex1 : MagnitudeAngleToComplex
  Mux1 : Mux
  Mux2 : Mux
  Terminator1 : Terminator
  Terminator2 : Terminator
  Trip : Outport  InitialOutput=0  VectorParamsAs1DForOutWhenUnconnected=on
  wires:
  Gain1/1 -> Comparing Current at Master Station/2
  " 1"/2 -> Mux2/1
  " 1"/4 -> Mux2/3
  " 1"/3 -> Mux2/2
  Mux2/1 -> Terminator2/1
  Gain/1 -> DAB8/1(a)
  Iremote/1 -> Gain/1
  " 1"/1 -> Demux2/1
  DAB8/1(d) -> " 1"/1
  Magnitude-Angle to Complex1/1 -> Comparision Scheme/2(I_Master)
  Demux2/2 -> Degrees to Radians/1
  Degrees to Radians/1 -> Magnitude-Angle to Complex1/2
  Demux2/1 -> Magnitude-Angle to Complex1/1
  " "/5 -> Mux1/4
  " "/4 -> Mux1/3
  " "/3 -> Mux1/2
  " "/2 -> Mux1/1
  Mux1/1 -> Terminator1/1
  " "/1 -> Demux1/1
  Comparision Scheme/1(Pickup) -> Trip/1
  DAB4/1(d) -> " "/1
  Ilocal/1 -> DAB4/1(a)
  Magnitude-Angle to Complex/1 -> Comparing Current at Master Station/1
  Icomp/1 -> Gain1/1
  Demux1/2 -> Degrees to Radians1/1
  Degrees to Radians1/1 -> Magnitude-Angle to Complex/2
  Comparing Current at Master Station/1 -> Comparision Scheme/1(I_Slave)
  " 1"/5 -> Mux2/4
  Demux1/1 -> Magnitude-Angle to Complex/1

== system Copy_4_of_baseModel/SM_WT1/Impedance Element 1/Impedance Relay Scheme/Analog filtering, signal conditioning ==
  note: Acquisition Block- analog filtering,
      | signal conditioning, sampling.
  Vin : Inport
  Iin : Inport  Port=2
  CURRENTS : Subsystem
  Mux{1..4} (4 alike) : Mux  Inputs=3
  VOLTAGES : Subsystem
  Vf : Outport  InitialOutput=0  VectorParamsAs1DForOutWhenUnconnected=on
  If : Outport  Port=2  InitialOutput=0  VectorParamsAs1DForOutWhenUnconnected=on
  If0 : Outport  Port=3  InitialOutput=0  VectorParamsAs1DForOutWhenUnconnected=on
  vf : Outport  Port=4  InitialOutput=0  VectorParamsAs1DForOutWhenUnconnected=on
  if : Outport  Port=5  InitialOutput=0  VectorParamsAs1DForOutWhenUnconnected=on
  wires:
  CURRENTS/4(k0I0f) -> If0/1
  Mux4/1 -> if/1
  Mux3/1 -> If/1
  CURRENTS/7(icf) -> Mux4/3
  CURRENTS/6(ibf) -> Mux4/2
  CURRENTS/5(iaf) -> Mux4/1
  CURRENTS/3(ICf) -> Mux3/3
  CURRENTS/2(IBf) -> Mux3/2
  CURRENTS/1(IAf) -> Mux3/1
  Iin/1 -> CURRENTS/1(Iabc)
  Mux2/1 -> vf/1
  VOLTAGES/6(vcf) -> Mux2/3
  VOLTAGES/5(vbf) -> Mux2/2
  VOLTAGES/4(vaf) -> Mux2/1
  VOLTAGES/3(VCf) -> Mux1/3
  VOLTAGES/2(VBf) -> Mux1/2
  VOLTAGES/1(VAf) -> Mux1/1
  Vin/1 -> VOLTAGES/1(Vabc)
  Mux1/1 -> Vf/1

== system Copy_4_of_baseModel/SM_WT1/Impedance Element 1/Impedance Relay Scheme/Combination of Voltages and Currents into 6 pairs (for each type of fault) ==
  note: Voltage and current combination block
  Vf : Inport
  If : Inport  Port=2
  If0 : Inport  Port=3
  "Currents Ia, Ib, Ic, kIo" : Demux  Outputs=3
  Ia+kIo : Sum  SaturateOnIntegerOverflow=on  InputSameDT=on  OutDataTypeStr=Inherit: Same as first input
  Ia-Ib : Sum  Inputs=+-  SaturateOnIntegerOverflow=on  InputSameDT=on  OutDataTypeStr=Inherit: Same as first input
  Ib+kIo : Sum  SaturateOnIntegerOverflow=on  InputSameDT=on  OutDataTypeStr=Inherit: Same as first input
  Ib-Ic : Sum  Inputs=+-  SaturateOnIntegerOverflow=on  InputSameDT=on  OutDataTypeStr=Inherit: Same as first input
  Ic+kIo : Sum  SaturateOnIntegerOverflow=on  InputSameDT=on  OutDataTypeStr=Inherit: Same as first input
  Ic-Ia : Sum  Inputs=+-  SaturateOnIntegerOverflow=on  InputSameDT=on  OutDataTypeStr=Inherit: Same as first input
  Mux{10..15} (6 alike) : Mux  Inputs=2
  Va-Vb : Sum  Inputs=+-  SaturateOnIntegerOverflow=on  InputSameDT=on  OutDataTypeStr=Inherit: Same as first input
  Vb-Vc : Sum  Inputs=+-  SaturateOnIntegerOverflow=on  InputSameDT=on  OutDataTypeStr=Inherit: Same as first input
  Vc-Va : Sum  Inputs=+-  SaturateOnIntegerOverflow=on  InputSameDT=on  OutDataTypeStr=Inherit: Same as first input
  "Voltages Va,Vb, Vc" : Demux  Outputs=3
  "Volt, Curr A-G" : Outport  InitialOutput=0  VectorParamsAs1DForOutWhenUnconnected=on
  "Volt, Curr B-G" : Outport  Port=2  InitialOutput=0  VectorParamsAs1DForOutWhenUnconnected=on
  "Volt, Curr C-G" : Outport  Port=3  InitialOutput=0  VectorParamsAs1DForOutWhenUnconnected=on
  "Volt, Curr B-C,B-C-G" : Outport  Port=4  InitialOutput=0  VectorParamsAs1DForOutWhenUnconnected=on
  "Volt, Curr C-A,C-A-G" : Outport  Port=5  InitialOutput=0  VectorParamsAs1DForOutWhenUnconnected=on
  "Volt, Curr A-B,A-B-C-G" : Outport  Port=6  InitialOutput=0  VectorParamsAs1DForOutWhenUnconnected=on
  wires:
  If0/1 -> Ib+kIo/2, Ia+kIo/2, Ic+kIo/2
  Mux13/1 -> "Volt, Curr B-C,B-C-G"/1
  Vb-Vc/1 -> Mux13/1
  Ib-Ic/1 -> Mux13/2
  Mux12/1 -> "Volt, Curr C-G"/1
  Ic+kIo/1 -> Mux12/2
  If/1 -> "Currents Ia, Ib, Ic, kIo"/1
  "Voltages Va,Vb, Vc"/3 -> Vc-Va/1, Vb-Vc/2, Mux12/1
  "Voltages Va,Vb, Vc"/2 -> Vb-Vc/1, Mux11/1, Va-Vb/2
  "Voltages Va,Vb, Vc"/1 -> Va-Vb/1, Mux10/1, Vc-Va/2
  Vf/1 -> "Voltages Va,Vb, Vc"/1
  Mux15/1 -> "Volt, Curr A-B,A-B-C-G"/1
  Mux14/1 -> "Volt, Curr C-A,C-A-G"/1
  Vc-Va/1 -> Mux14/1
  Mux11/1 -> "Volt, Curr B-G"/1
  Mux10/1 -> "Volt, Curr A-G"/1
  Ia+kIo/1 -> Mux10/2
  Ib+kIo/1 -> Mux11/2
  Ic-Ia/1 -> Mux14/2
  Va-Vb/1 -> Mux15/1
  Ia-Ib/1 -> Mux15/2
  "Currents Ia, Ib, Ic, kIo"/2 -> Ia-Ib/2, Ib-Ic/1, Ib+kIo/1
  "Currents Ia, Ib, Ic, kIo"/3 -> Ic-Ia/1, Ib-Ic/2, Ic+kIo/1
  "Currents Ia, Ib, Ic, kIo"/1 -> Ia-Ib/1, Ic-Ia/2, Ia+kIo/1

== system Copy_4_of_baseModel/SM_WT1/Impedance Element 1/Impedance Relay Scheme/Fault A-B-C Measurement ==
  A-B-C : Inport
  <V : Inport  Port=2
  Complex to Real-Imag : ComplexToRealImag
  Impedance Module : Product  Inputs=*/  SaturateOnIntegerOverflow=on  RndMeth=Zero  InputSameDT=on  OutDataTypeStr=Inherit: Same as first input
  Mux{,1..4} (5 alike) : Mux  Inputs=2
  Voltage Current : Demux  Outputs=2
  Zone 1 : Subsystem  mask(Zone){Xr=ZoneImpedance(1)*sin(LineAngle*pi/180), Rr=ZoneImpedance(1)*cos(LineAngle*pi/180), Td=ZoneTime(1)}
      mask prompts: Xr "Reactance reach [ohm]"; Rr "Resistance reach [ohm]"; Td "Time delay [s]"
  Zone 2 : Subsystem  mask(Zone){Xr=ZoneImpedance(2)*sin(LineAngle*pi/180), Rr=ZoneImpedance(2)*cos(LineAngle*pi/180), Td=ZoneTime(2)}
      mask prompts: Xr "Reactance reach [ohm]"; Rr "Resistance reach [ohm]"; Td "Time delay [s]"
  Zone 3 : Subsystem  mask(Zone){Xr=ZoneImpedance(3)*sin(LineAngle*pi/180), Rr=ZoneImpedance(3)*cos(LineAngle*pi/180), Td=ZoneTime(3)}
      mask prompts: Xr "Reactance reach [ohm]"; Rr "Resistance reach [ohm]"; Td "Time delay [s]"
  Zone 4 : Subsystem  mask(Zone){Xr=ZoneImpedance(4)*sin(LineAngle*pi/180), Rr=ZoneImpedance(4)*cos(LineAngle*pi/180), Td=ZoneTime(4)}
      mask prompts: Xr "Reactance reach [ohm]"; Rr "Resistance reach [ohm]"; Td "Time delay [s]"
  Zone1Z : Terminator
  Zone2Z : Terminator
  Zone3Z : Terminator
  Zone4Z : Terminator
  Zone1 : Outport  InitialOutput=0  VectorParamsAs1DForOutWhenUnconnected=on
  Zone2 : Outport  Port=2  InitialOutput=0  VectorParamsAs1DForOutWhenUnconnected=on
  Zone3 : Outport  Port=3  InitialOutput=0  VectorParamsAs1DForOutWhenUnconnected=on
  Zone4 : Outport  Port=4  InitialOutput=0  VectorParamsAs1DForOutWhenUnconnected=on
  wires:
  A-B-C/1 -> Voltage Current/1
  Mux/1 -> Zone 1/1(Z), Zone 3/1(Z), Zone 4/1(Z), Zone 2/1(Z)
  Zone 1/1(TRIP) -> Zone1/1
  Zone 1/2(Zm) -> Mux1/1
  Zone 1/3(Zr) -> Mux1/2
  Zone 2/2(Zm) -> Mux2/1
  Zone 2/3(Zr) -> Mux2/2
  Zone 3/2(Zm) -> Mux3/1
  Zone 3/3(Zr) -> Mux3/2
  Zone 4/2(Zm) -> Mux4/1
  Zone 4/3(Zr) -> Mux4/2
  Zone 2/1(TRIP) -> Zone2/1
  Zone 3/1(TRIP) -> Zone3/1
  Zone 4/1(TRIP) -> Zone4/1
  Complex to Real-Imag/1 -> Mux/1
  Complex to Real-Imag/2 -> Mux/2
  <V/1 -> Zone 1/2(<V), Zone 2/2(<V), Zone 3/2(<V), Zone 4/2(<V)
  Mux1/1 -> Zone1Z/1
  Mux2/1 -> Zone2Z/1
  Mux3/1 -> Zone3Z/1
  Mux4/1 -> Zone4Z/1
  Impedance Module/1 -> Complex to Real-Imag/1
  Voltage Current/1 -> Impedance Module/1
  Voltage Current/2 -> Impedance Module/2

== system Copy_4_of_baseModel/SM_WT1/Impedance Element 1/Impedance Relay Scheme/Fault A-G Measurement ==
  A-G : Inport
  <V : Inport  Port=2
  Complex to Real-Imag : ComplexToRealImag
  Impedance Module : Product  Inputs=*/  SaturateOnIntegerOverflow=on  RndMeth=Zero  InputSameDT=on  OutDataTypeStr=Inherit: Same as first input
  Mux{,1..4} (5 alike) : Mux  Inputs=2
  Voltage Current : Demux  Outputs=2
  Zone 1 : Subsystem  mask(Zone){Xr=ZoneImpedance(1)*sin(LineAngle*pi/180), Rr=ZoneImpedance(1)*cos(LineAngle*pi/180), Td=ZoneTime(1)}
      mask prompts: Xr "Reactance reach [ohm]"; Rr "Resistance reach [ohm]"; Td "Time delay [s]"
  Zone 2 : Subsystem  mask(Zone){Xr=ZoneImpedance(2)*sin(LineAngle*pi/180), Rr=ZoneImpedance(2)*cos(LineAngle*pi/180), Td=ZoneTime(2)}
      mask prompts: Xr "Reactance reach [ohm]"; Rr "Resistance reach [ohm]"; Td "Time delay [s]"
  Zone 3 : Subsystem  mask(Zone){Xr=ZoneImpedance(3)*sin(LineAngle*pi/180), Rr=ZoneImpedance(3)*cos(LineAngle*pi/180), Td=ZoneTime(3)}
      mask prompts: Xr "Reactance reach [ohm]"; Rr "Resistance reach [ohm]"; Td "Time delay [s]"
  Zone 4 : Subsystem  mask(Zone){Xr=ZoneImpedance(4)*sin(LineAngle*pi/180), Rr=ZoneImpedance(4)*cos(LineAngle*pi/180), Td=ZoneTime(4)}
      mask prompts: Xr "Reactance reach [ohm]"; Rr "Resistance reach [ohm]"; Td "Time delay [s]"
  Zone1Z : Terminator
  Zone2Z : Terminator
  Zone3Z : Terminator
  Zone4Z : Terminator
  Zone1 : Outport  InitialOutput=0  VectorParamsAs1DForOutWhenUnconnected=on
  Zone2 : Outport  Port=2  InitialOutput=0  VectorParamsAs1DForOutWhenUnconnected=on
  Zone3 : Outport  Port=3  InitialOutput=0  VectorParamsAs1DForOutWhenUnconnected=on
  Zone4 : Outport  Port=4  InitialOutput=0  VectorParamsAs1DForOutWhenUnconnected=on
  wires:
  Voltage Current/2 -> Impedance Module/2
  Voltage Current/1 -> Impedance Module/1
  Impedance Module/1 -> Complex to Real-Imag/1
  Mux4/1 -> Zone4Z/1
  Mux3/1 -> Zone3Z/1
  Mux2/1 -> Zone2Z/1
  Mux1/1 -> Zone1Z/1
  <V/1 -> Zone 4/2(<V), Zone 3/2(<V), Zone 2/2(<V), Zone 1/2(<V)
  Complex to Real-Imag/2 -> Mux/2
  Complex to Real-Imag/1 -> Mux/1
  Zone 4/1(TRIP) -> Zone4/1
  Zone 3/1(TRIP) -> Zone3/1
  Zone 2/1(TRIP) -> Zone2/1
  Zone 4/3(Zr) -> Mux4/2
  Zone 4/2(Zm) -> Mux4/1
  Zone 3/3(Zr) -> Mux3/2
  Zone 3/2(Zm) -> Mux3/1
  Zone 2/3(Zr) -> Mux2/2
  Zone 2/2(Zm) -> Mux2/1
  Zone 1/3(Zr) -> Mux1/2
  Zone 1/2(Zm) -> Mux1/1
  Zone 1/1(TRIP) -> Zone1/1
  Mux/1 -> Zone 2/1(Z), Zone 4/1(Z), Zone 3/1(Z), Zone 1/1(Z)
  A-G/1 -> Voltage Current/1
